simulink model "WS_20_Nils_Bestehorn_modell"  (R2021b)
settings: Solver=FixedStepAuto  StartTime=0.0  StopTime=6  FixedStep=0.01  RelTol=1e-3
values from neighbouring files (symbols this model uses):
  c = 5000    [WS_20_Nils_Bestehorn_mfile.m]
  d = 4    [WS_20_Nils_Bestehorn_mfile.m]
  g = 9.81    [WS_20_Nils_Bestehorn_mfile.m]
  iG = 10    [WS_20_Nils_Bestehorn_mfile.m]
  Jm = 0.5    [WS_20_Nils_Bestehorn_mfile.m]
  JTm = 5    [WS_20_Nils_Bestehorn_mfile.m]
  LM = 0.1    [WS_20_Nils_Bestehorn_mfile.m]
  m = 40    [WS_20_Nils_Bestehorn_mfile.m]
  ML = m*g*r    (= 98.1)    [WS_20_Nils_Bestehorn_mfile.m]
  phii = 2    [WS_20_Nils_Bestehorn_mfile.m]
  phiM = 0.9    [WS_20_Nils_Bestehorn_mfile.m]
  r = 250*10^-3    (= 0.25)    [WS_20_Nils_Bestehorn_mfile.m]
  RM = 1    [WS_20_Nils_Bestehorn_mfile.m]
  Uqmax = 240    [WS_20_Nils_Bestehorn_mfile.m]
undefined symbols (not defined in the file or in its folder): sigbuilder_block
settings Model: Creator=nilsb  LastModifiedBy=nilsb

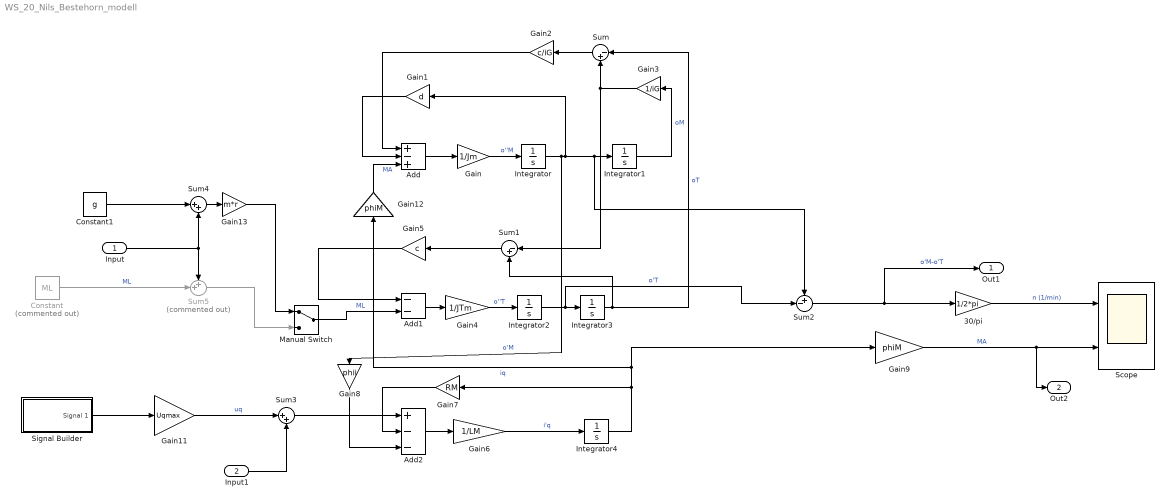
== system WS_20_Nils_Bestehorn_modell ==
  Input : Inport
  Input1 : Inport  Port=2
  30/pi : Gain  Gain=1/2*pi
  Add : Sum  Inputs=+-+
  Add1 : Sum  Inputs=--
  Add2 : Sum  Inputs=+--
  Constant : Constant  Commented=on  Value=ML
  Constant1 : Constant  Value=g
  Gain : Gain  Gain=1/Jm
  Gain1 : Gain  Gain=d
  Gain11 : Gain  Gain=Uqmax
  Gain12 : Gain  Gain=phiM
  Gain13 : Gain  Gain=m*r
  Gain2 : Gain  Gain=c/iG
  Gain3 : Gain  Gain=1/iG
  Gain4 : Gain  Gain=1/JTm
  Gain5 : Gain  Gain=c
  Gain6 : Gain  Gain=1/LM
  Gain7 : Gain  Gain=RM
  Gain8 : Gain  Gain=phii
  Gain9 : Gain  Gain=phiM
  Integrator{,1..4} (5 alike) : Integrator
  Manual Switch : ManualSwitch
  Scope : Scope  NumInputPorts=2
  Signal Builder : Subsystem  Tag=STV Subsys  LoadFcn=sigbuilder_block('load');  StartFcn=sigbuilder_block('start');  StopFcn=sigbuilder_block('stop');  ClipboardFcn=sigbuilder_block('clipboard');  mask(Sigbuilder block){tuvar=[0:10]}
      mask help: Simulink:masks:SigbuilderBlock_MD
      mask init:
      | if ~strcmp(get_param(bdroot(gcbh),'SimulationStatus'),'stopped') tuvar = sigbuilder_block('maskInit'); end
      settings: CopyFcn=sigbuilder_block('copy');  DeleteFcn=sigbuilder_block('delete');  ModelCloseFcn=sigbuilder_block('modelClose');  PreSaveFcn=sigbuilder_block('preSave');  PauseFcn=sigbuilder_block('pause');  ContinueFcn=sigbuilder_block('continue');  NameChangeFcn=sigbuilder_block('namechange');  OpenFcn=sigbuilder_block('open',[437.6 199.2 550.4 400 ]);  CloseFcn=sigbuilder_block('close');
      mask Display: plot(0, 0, 100, 100,[2, 2, 32, 32, 2], [68, 8, 8, 68, 68],[32, 2], [38, 38], [32, 19, 2],[53, 60, 44], [32, 17, 17, 2],[16, 16, 31, 31]);txt = getActiveGroup(gcbh);text(2, 100, txt,'verticalAlignment', 'top');
  Sum : Sum  Inputs=|-+
  Sum1 : Sum  Inputs=|-+
  Sum2 : Sum  Inputs=+-|
  Sum3 : Sum  Inputs=|++
  Sum4 : Sum  Inputs=|++
  Sum5 : Sum  Commented=on  Inputs=++|
  Out1 : Outport
  Out2 : Outport  Port=2
  wires:
  Integrator/1 -> Gain8/1, Gain1/1, Sum2/1, Integrator1/1  "o'M"
  Gain/1 -> Integrator/1  "o''M"
  Integrator1/1 -> Gain3/1  "oM"
  Add/1 -> Gain/1
  Gain2/1 -> Add/1
  Gain1/1 -> Add/2
  Sum/1 -> Gain2/1
  Gain3/1 -> Sum1/1, Sum/2
  Integrator3/1 -> Sum/1, Sum1/2  "oT"
  Gain12/1 -> Add/3  "MA"
  Integrator2/1 -> Sum2/2, Integrator3/1  "o'T"
  Gain4/1 -> Integrator2/1  "o''T"
  Add1/1 -> Gain4/1
  Constant/1 -> Sum5/2  "ML"
  Gain5/1 -> Add1/1
  Sum1/1 -> Gain5/1
  Integrator4/1 -> Gain12/1, Gain9/1, Gain7/1  "iq"
  Gain6/1 -> Integrator4/1  "i'q"
  Add2/1 -> Gain6/1
  Gain11/1 -> Sum3/1  "uq"
  Gain7/1 -> Add2/2
  Gain8/1 -> Add2/3
  30/pi/1 -> Scope/1  "n (1/min)"
  Gain9/1 -> Out2/1, Scope/2  "MA"
  Sum2/1 -> 30/pi/1, Out1/1  "o'M-o'T"
  Signal Builder/1(Signal 1) -> Gain11/1
  Sum3/1 -> Add2/1
  Input1/1 -> Sum3/2
  Gain13/1 -> Manual Switch/1
  Constant1/1 -> Sum4/1
  Sum4/1 -> Gain13/1
  Input/1 -> Sum5/1, Sum4/2
  Manual Switch/1 -> Add1/2  "ML"
  Sum5/1 -> Manual Switch/2

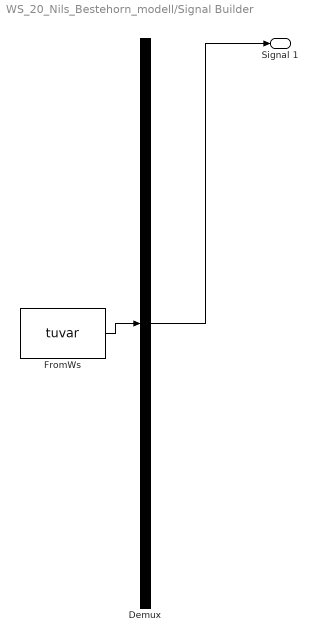
== system WS_20_Nils_Bestehorn_modell/Signal Builder ==
  Demux : Demux  Tag=STV Demux  Outputs=1
      settings: DisplayOption=none
  FromWs : FromWorkspace  Tag=STV FromWs  VariableName=tuvar
      SigBuilderData=|
      | common.afterFinalStr = 'Extrapolate'
      | common.sampleTime = 0
      | dataSet.timeRange = [0 10]
      | dataSet.name = 'Group 1'
      | sbobj.Groups.Name = 'Group 1'
      | sbobj.Groups.Signals.Name = 'Signal 1'
      | sbobj.Groups.Signals.XData = [0 0.2 4 4 10]
      | sbobj.Groups.Signals.YData = [0 1 1 0.4 0.4]
  Signal 1 : Outport  Tag=STV Outport
  wires:
  Demux/1 -> Signal 1/1
  FromWs/1 -> Demux/1
